simulink model "P3P_Grunert"  (R2023b)
settings: Solver=FixedStepDiscrete  StartTime=0.0  StopTime=0  RelTol=1e-3
values from neighbouring files (symbols this model uses):
  checkerSize = [5, 8]    [P3P_processVideo.m]
  checkerSquareLength = 31    [P3P_processVideo.m]
  I_current = I_allFrames(:,:,q)    [P3P_processVideo.m]
  K = [1109 0 640; 0 1109 360; 0 0 1]    [P3P_processVideo.m]
  x_pnts_i = round(x_pnts_i)    [P3P_processVideo.m]
  X_pnts_w = calcCheckerEdgeCoords_w(checkerSize, checkerSquareLength)    [P3P_processVideo.m]
undefined symbols (not defined in the file or in its folder): gray, Rec, SDTV
libraries: dspinverses x5, dspmathops x5, visiontextngfix x4, matrix_library x2, visionconversions x1, visionanalysis x1, dspvision x1, visionsources x1
(part 2 of 3)

== matlab function P3P_Grunert/While Iterator Subsystem/Perform P3P and RANSAC on checkerboard/Custom P3P solver (Grunert)/Find ray lengths jingnanshi convention ==
  data: l_AB input; soln output size=[4, 3]; l_BC input; l_AC input; theta input
function soln = fcn(l_AB, l_BC, l_AC, theta)

soln = zeros(4, 3);


%Calculate polynomial coefficients
a = l_AC;
b = l_BC;
c = l_AB;

gamma = theta(1); %theta_AB
alpha = theta(3); %theta_AC
beta = theta(2); %theta_BC


a2minc2ovb2 =  (a^2 - c^2) / b^2 ;
a2plusc2ovb2 =  (a^2 + c^2) / b^2; 


A0 = (1 + a2minc2ovb2)^2   -   4*((a*cos(gamma)/b)^2);
A1 = - a2minc2ovb2 * (1 + a2minc2ovb2) * cos(beta)     +    2 * ((a * cos(gamma) /  b)^2) * cos (beta)     -     (1 - a2plusc2ovb2) * cos(alpha) * cos(gamma);
A1 = 4 * A1;
A2 = a2minc2ovb2^2   -   1   +   2*((a2minc2ovb2 * cos(beta))^2)  +  2 *(  ((b^2 - c^2)/(b^2))  * (cos(alpha))^2  )   - 4*a2plusc2ovb2*cos(alpha)*cos(beta)*cos(gamma)   +   2*((b^2 - a^2)/(b^2))*((cos(gamma))^2);
A2 = 2* A2;
A3 = a2minc2ovb2 * (1 - a2minc2ovb2) * cos(beta)    -   (1 - a2plusc2ovb2) * cos(alpha) * cos(gamma)    +   2 * ((c * cos(alpha)/b)^2) * cos(beta);
A3 = 4 * A3;
A4 = (a2minc2ovb2 -1)^2   - (2 * c * cos(alpha) / b)^2;

%Solve polynomial
%instead of u and v for polynomial, use g and h - i.e., g = s2/s1 and h =
%s3/s1
p = [A4 A3 A2 A1 A0];
h = roots(p);
%choose only real roots - maybe this is not necessary?
h = h(imag(h)==0);
h = real(h);

%%%%%%%%%%%%%%%%%%%%%%%%%%%%%%%%%%%%%%%%%
%%%%%%%%%%%%%Find ray lengths

%For s1, which corresponds to sB. Should end up with 4 solns
%s_A =    (b^2) / (1 + h.^2  +  2*h*cos(beta)  )     ;
%s_A = s_A(s_A~=0);
%s_A = transpose(s_A);
%s_A = s_A.^0.5;


%Find s2, which corresponds to sC.
counter = 1
for i = 1:numel(h)

    s_1 = (b^2) / (1 + (h(i)^2) - 2*h(i)*cos(beta));
    s_1 = sqrt(s_1);

    G2 = s_1^2;
    G1 = - 2 * (s_1^2) * cos(gamma);
    G0 = (s_1^2 -c^2);

    g = roots([G2 G1 G0]);
    g = g(imag(g)==0);
    g = real(g);

    %First, solve for s_C, since it only depends on h and s_A:

    for j = 1:numel(g)
        soln(counter, 1) = s_1 * g(j);
        soln(counter, 3) = s_1 * h(i);
        soln(counter, 2) = s_1; 
        counter = counter +1
    end

end

== matlab function P3P_Grunert/While Iterator Subsystem/Perform P3P and RANSAC on checkerboard/Custom P3P solver (Grunert)/MATLAB Function4 ==
  data: pnts_vectorsCameraCoords input; theta_raysABC_radians output
function theta_raysABC_radians = calcProjectionRayAngles(pnts_vectorsCameraCoords)

A_x_c = pnts_vectorsCameraCoords(:,1);
B_x_c = pnts_vectorsCameraCoords(:,2);
C_x_c = pnts_vectorsCameraCoords(:,3);

%theta_AB = acos(dot(A_x_c, B_x_c));
%theta_BC = acos(dot(B_x_c, C_x_c));
%theta_AC = acos(dot(C_x_c, A_x_c));

%theta_AB = atan2(norm(cross(A_x_c, B_x_c)), dot(A_x_c, B_x_c));
%theta_BC = atan2(norm(cross(B_x_c, C_x_c)), dot(B_x_c, C_x_c));
%theta_AC = atan2(norm(cross(A_x_c, C_x_c)), dot(A_x_c, C_x_c)); 

theta_AB = acos(dot(A_x_c, B_x_c)/(norm(A_x_c)*norm(B_x_c)));
theta_BC = acos(dot(B_x_c, C_x_c)/(norm(B_x_c)*norm(C_x_c)));
theta_AC = acos(dot(A_x_c, C_x_c)/(norm(A_x_c)*norm(C_x_c)));


theta_raysABC_radians = [theta_AB; theta_BC; theta_AC];

== matlab function P3P_Grunert/While Iterator Subsystem/Perform P3P and RANSAC on checkerboard/Detect checkerboard corners ==
  data: x_pts_i output size=[60, 2]; I input; checkerSize output size=[1, 2]
function [x_pts_i, checkerSize]= findCheckerboardPnts(I)

%I = imread(fullfile('C:\Users\Alyssa\OneDrive - University of Cape Town\Vision\ESP32-CAM\CamCalibrationPics', '1.jpg'));
Points = detectCheckerboardPoints(I);
[~,checkerSize] = detectCheckerboardPoints(I);
x_pts_i = round(Points);
%checkerSize = Size;
%checkerPoints = imagePoints;

== matlab function P3P_Grunert/While Iterator Subsystem/Perform P3P and RANSAC on checkerboard/Extract best Rte (most inliers) ==
  data: Rte input; bestRt output; bestRt_error output; bestRt_inliers output
function [bestRt, bestRt_error, bestRt_inliers]= fcn(Rte)
%Function looks through 3-dim array Rte to find the Rt that has the highest
%number of inliers. This is output as the "best" Rt


index_bestRte = 0;
mostInliers = 0;

for n=1: size(Rte, 3)

    if Rte(1, 5, n) > mostInliers
        mostInliers = Rte(1, 5, n);
        index_bestRte = n;
    end
end

bestRt = Rte(:, 1:4, index_bestRte);
bestRt_error = Rte(2, 5, index_bestRte);
bestRt_inliers = Rte(1, 5, index_bestRte);

== matlab function P3P_Grunert/While Iterator Subsystem/Perform P3P and RANSAC on checkerboard/For Each Subsystem/Choose best solutiion from iteration ==
  data: Rt input; mostInliers_Rt output size=[3,4]; x_rem_i input; X_rem_w input; mostInliers output; Inlier_threshold input; mostInliers_avgError output; K input
function [mostInliers_Rt, mostInliers, mostInliers_avgError] = fcn(Rt, x_rem_i, X_rem_w, Inlier_threshold, K)
%This function finds the best Rt (transformation matrix) from the current
%RANSAC iteration. Here, "best" means "most inliers". I.e., for each 
%possible Rt out of the P3P solver, each of the remaining detected corners are 
%reprojected (using this Rt). If the reprojection error for a given point
%is below a certain threshold, it is considered an inlier. 
%Out of the 4 possible Rts for each P3P iteration, only that with the
%highest number of iterations will be passed out of this function.

%for each possible solution given by the P3P solver
numTestPts =  size(x_rem_i, 1);
mostInliers = 0;
mostInliers_Rt = zeros(3, 4);
mostInliers_avgError = 0;

for n = 1: size(Rt, 3)

    
    numInliers_n = 0;
    avgError_n = 0;

    %calculate reprojection error 
    for j = 1: numTestPts

        X_j_w = transpose(X_rem_w(j, :));
        x_j_i_real = transpose(x_rem_i(j,:));
        x_j_i_proj = zeros(2, 1);
        x_j_i_proj_homo = zeros(3,1);

        %project point (in homogenous coordinates)
        x_j_i_proj_homo = K * (  (Rt(:, 1:3, n) * X_j_w)  + Rt(:, 4,n)  );

        %Normalise by the 3rd dimension
        x_j_i_proj(1) = x_j_i_proj_homo(1)/x_j_i_proj_homo(3);
        x_j_i_proj(2) = x_j_i_proj_homo(2)/x_j_i_proj_homo(3);

        %calculate reprojection error for current point
        error_j = norm(x_j_i_proj - x_j_i_real);
        avgError_n = avgError_n + error_j;

        %check if an inlier
        if error_j < Inlier_threshold
            numInliers_n = numInliers_n + 1;
        end
    end
    
    %Calculate mean error (could be useful)
    avgError_n = avgError_n / numTestPts;

    %If current Rt achieves more inliers than previous best, then update
    %"best"
    if numInliers_n > mostInliers
        mostInliers = numInliers_n;
        mostInliers_avgError = avgError_n;
        mostInliers_Rt = Rt(:, :, n);
    end
end

== matlab function P3P_Grunert/While Iterator Subsystem/Perform P3P and RANSAC on checkerboard/For Each Subsystem/Create array ==
  data: Rte_n output size=[3,5]; mostInliers_Rt input; mostInliers input; mostInliers_avgError input
function Rte_n = fcn(mostInliers_Rt, mostInliers, mostInliers_avgError)

Rte_n = zeros(3, 5);
Rte_n(:, 1:4) = mostInliers_Rt;
Rte_n(1, 5) = mostInliers;
Rte_n(2, 5) = mostInliers_avgError;

== matlab function P3P_Grunert/While Iterator Subsystem/Perform P3P and RANSAC on checkerboard/For Each Subsystem/Custom P3P solver (Grunert)/Calc lengths of triangle sides (world frame) ==
  data: X_ABC_w input; l_AB output; l_BC output; l_AC output
function [l_AB, l_BC, l_AC]= fcn(X_ABC_w)

l_AB = norm(X_ABC_w(:,1)-X_ABC_w(:,2));
l_AC = norm(X_ABC_w(:,1)-X_ABC_w(:,3));
l_BC = norm(X_ABC_w(:,2)-X_ABC_w(:,3));

== matlab function P3P_Grunert/Subsystem/Custom P3P solver (Kneip)/Invert Rt (swap coord transformation)1 ==
  data: Rt input; Rt_converted output size=[3,4]
function Rt_converted = fcn(Rt)

R_inv = zeros(3,3);
t_inv = zeros(3,1);

R = Rt(1:3, 1:3);
t = Rt(1:3, 4);
  
R_inv(1:3, 1:3) = transpose(R);
t_inv = - R_inv * t;

%R_matlab_W = [-1 0 0; 0 1 0; 0 0 1];
%R_matlab_W = [-1 0 0; 0 -1 0; 0 0 1];
%R_conv = R_matlab_W * R_inv;
%t_conv = R_matlab_W * t_inv;

Rt_converted = [R_inv t_inv];

== matlab function P3P_Grunert/Subsystem/Custom P3P solver (Grunert)/Calculate rotation matrix and translation vector using SVD ==
  data: X_ABC_w input; Rt output size=[3,4,8]; X_ABC_c input
function Rt = fcn(X_ABC_w, X_ABC_c)

%We have 3 points in the world frame and in the camera frame. Now we need 
%to find the rotation and translation matrices that would convert one to 
%the other.
%This is the classic Procrustes problem, which we can solve using singular 
%value decomposition. We will end up with one rotation matrix and one
%translation vector for each of the possible sets of coordinates. 

 R = zeros(3,3,8);
 t = zeros(3,8);
 Rt = zeros(3,4,8);

 P = X_ABC_w;
 %Find the mean of the columns (i.e. the centroid of the shape)
 P_centroid = mean(P,2);
 %Centre each vector
 Q = P - P_centroid;

%for each possible solution
for i=1: size(X_ABC_c, 3)

    %Condition each vector as above
    P_dash =  X_ABC_c(:, :, i);
    P_dash_centroid = mean(P_dash, 2);
    Q_dash = P_dash - P_dash_centroid;
    
    %Find the covariance matrix
    H = Q_dash * transpose(Q);

    %Perform SVD (singular value decomposition)
    [U, S, V] = svd(H);

    % %Calculate rotation matrix
    R(:,:,i) = U * transpose(V);
    %Correct sign if needed
    if det(R(:,:,i))<0
        U(:,end) = -1 * U(:,end);
        %and recompute R
        R(:, :, i) = U * transpose(V);
    end

    % R(:,:,i) = transpose(U) * V;
    % if det(R(:,:,i)) < 0
    %     V(:,end) = -V(:,end);
    %     R = transpose(U) * V;
    % end

    %Calculate the translation vector:
    t(:, i) = P_dash_centroid - R(:, :, i)*P_centroid;

    Rt(:,:, i)= [R(:,:,i) t(:, i)];

end

== matlab function P3P_Grunert/While Iterator Subsystem/Perform P3P and RANSAC on checkerboard/For Each Subsystem/Custom P3P solver (Grunert)/Calculate rotation matrix and translation vector using SVD ==
  data: X_ABC_w input; Rt output size=[3,4,8]; X_ABC_c input
function Rt = fcn(X_ABC_w, X_ABC_c)

%We have 3 points in the world frame and in the camera frame. Now we need 
%to find the rotation and translation matrices that would convert one to 
%the other.
%This is the classic Procrustes problem, which we can solve using singular 
%value decomposition. We will end up with one rotation matrix and one
%translation vector for each of the possible sets of coordinates. 

 R = zeros(3,3,8);
 t = zeros(3,8);
 Rt = zeros(3,4,8);

 P = X_ABC_w;
 %Find the mean of the columns (i.e. the centroid of the shape)
 P_centroid = mean(P,2);
 %Centre each vector
 Q = P - P_centroid;

%for each possible solution
for i=1: size(X_ABC_c, 3)

    %Condition each vector as above
    P_dash =  X_ABC_c(:, :, i);
    P_dash_centroid = mean(P_dash, 2);
    Q_dash = P_dash - P_dash_centroid;
    
    %Find the covariance matrix
    H = Q_dash * transpose(Q);

    %Perform SVD (singular value decomposition)
    [U, S, V] = svd(H);

    %Calculate rotation matrix
    R(:,:,i) = U * transpose(V);
    %Correct sign if needed
    if det(R(:,:,i))<0
        U(:,end) = U(:,end) * (-1);
        %and recompute R
        R(:, :, i) = U * transpose(V);
    end

    %Calculate the translation vector:
    t(:, i) = P_dash_centroid - R(:, :, i)*P_centroid;

    Rt(:,:, i)= [R(:,:,i) t(:, i)];

end

== matlab function P3P_Grunert/Subsystem/Custom P3P solver (Kneip)/Invert Rt (swap coord transformation)2 ==
  data: Rt input; Rt_converted output size=[3,4]
function Rt_converted = fcn(Rt)

R_inv = zeros(3,3);

R = Rt(1:3, 1:3);
t = Rt(1:3, 4);
  
R_inv(1:3, 1:3) = transpose(R);
t_inv = - R_inv * t;

%R_matlab_W = [-1 0 0; 0 1 0; 0 0 1];
%R_matlab_W = [-1 0 0; 0 -1 0; 0 0 1];
%R_conv = R_matlab_W * R_inv;
%t_conv = R_matlab_W * t_inv;

Rt_converted = [R_inv t_inv];

== matlab function P3P_Grunert/While Iterator Subsystem/Perform P3P and RANSAC on checkerboard/For Each Subsystem/Custom P3P solver (Grunert)/Compute 3D coords of control points A, B, C in camera coord system ==
  data: s_ABC input; X_c_ABC output size=[3,3,8]; x_c_norm_ABC input
function X_c_ABC = fcn(s_ABC, x_c_norm_ABC)
    X_c_ABC = zeros(3,3,8);


    %For each combination of possible lengths
    for n=1:size(s_ABC, 1)
        %Get the vector between the camera and the point by multiplying
        %each element of the (unit) direction vector with the associated
        %ray length from the solution. 
        %The solution takes the form: [s_A1 s_B1 s_C1; s_A2 sB2...].
        %The direction vectors take the form: [xA xB xC; yA yB...].
        X_c_ABC(:, 1, n) = s_ABC(n, 1) * x_c_norm_ABC(:, 1);
        X_c_ABC(:, 2, n) = s_ABC(n, 2) * x_c_norm_ABC(:, 2);
        X_c_ABC(:, 3, n) = s_ABC(n, 3) * x_c_norm_ABC(:, 3);
    end

== matlab function P3P_Grunert/While Iterator Subsystem/Perform P3P and RANSAC on checkerboard/For Each Subsystem/Custom P3P solver (Grunert)/Find ray lengths ==
  data: l_AB input; soln output size=[4, 3]; l_BC input; l_AC input; theta input
function soln = fcn(l_AB, l_BC, l_AC, theta)

soln = zeros(4, 3);


%Calculate polynomial coefficients
a = l_BC;
b = l_AC;
c = l_AB;

gamma = theta(3); %theta_AC
alpha = theta(2); %theta_BC
beta = theta(1); %theta_AB


a2minc2ovb2 =  (a^2 - c^2) / b^2 ;
a2plusc2ovb2 =  (a^2 + c^2) / b^2; 


A0 = (1 + a2minc2ovb2)^2   -   4*((a*cos(gamma)/b)^2);
A1 = - a2minc2ovb2 * (1 + a2minc2ovb2) * cos(beta)     +    2 * ((a * cos(gamma) /  b)^2) * cos (beta)     -     (1 - a2plusc2ovb2) * cos(alpha) * cos(gamma);
A1 = 4 * A1;
A2 = a2minc2ovb2^2   -   1   +   2*((a2minc2ovb2 * cos(beta))^2)  +  2 *(  ((b^2 - c^2)/(b^2))  * (cos(alpha))^2  )   - 4*a2plusc2ovb2*cos(alpha)*cos(beta)*cos(gamma)   +   2*((b^2 - a^2)/(b^2))*(cos(gamma)^2);
A2 = 2* A2;
A3 = a2minc2ovb2 * (1 - a2minc2ovb2) * cos(beta)    -   (1 - a2plusc2ovb2) * cos(alpha) * cos(gamma)    +   2 * ((c * cos(alpha)/b)^2) * cos(beta);
A3 = 4 * A3;
A4 = (a2minc2ovb2 -1)^2   - (2 * c * cos(alpha) / b)^2;

%Solve polynomial
%instead of u and v for polynomial, use g and h - i.e., g = s2/s1 and h =
%s3/s1
p = [A4 A3 A2 A1 A0];
h = roots(p);
%choose only real roots - maybe this is not necessary?
h = h(imag(h)==0);
h = real(h);

%%%%%%%%%%%%%%%%%%%%%%%%%%%%%%%%%%%%%%%%%
%%%%%%%%%%%%%Find ray lengths

%For s1, which corresponds to sA. Should end up with 4 solns
%s_A =    (b^2) / (1 + h.^2  +  2*h*cos(beta)  )     ;
%s_A = s_A(s_A~=0);
%s_A = transpose(s_A);
%s_A = s_A.^0.5;


%Find s2, which corresponds to sC.
counter = 1
for i = 1:numel(h)

    s_A = (b^2) / (1 + (h(i)^2) - 2*h(i)*cos(beta));
    s_A = sqrt(s_A);

    G2 = s_A^2;
    G1 = - 2 * (s_A^2) * cos(gamma);
    G0 = (s_A -c)^2;

    g = roots([G2 G1 G0]);
    g = g(imag(g)==0);
    g = real(g);

    %First, solve for s_C, since it only depends on h and s_A:

    for j = 1:numel(g)
        soln(counter, 1) = s_A;
        soln(counter, 3) = s_A * g(j);
        soln(counter, 2) = h(i) * s_A;
        counter = counter +1
    end

end

== matlab function P3P_Grunert/While Iterator Subsystem/Perform P3P and RANSAC on checkerboard/For Each Subsystem/Custom P3P solver (Grunert)/Find ray lengths jingnanshi convention ==
  data: l_AB input; soln output size=[8, 3]; l_BC input; l_AC input; theta input
function soln = fcn(l_AB, l_BC, l_AC, theta)

soln = zeros(8, 3);


%Calculate polynomial coefficients
a = l_AC;
b = l_BC;
c = l_AB;

gamma = theta(1); %theta_AB
alpha = theta(3); %theta_AC
beta = theta(2); %theta_BC


a2minc2ovb2 =  (a^2 - c^2) / b^2 ;
a2plusc2ovb2 =  (a^2 + c^2) / b^2; 


A0 = (1 + a2minc2ovb2)^2   -   4*((a*cos(gamma)/b)^2);
A1 = - a2minc2ovb2 * (1 + a2minc2ovb2) * cos(beta)     +    2 * ((a * cos(gamma) /  b)^2) * cos (beta)     -     (1 - a2plusc2ovb2) * cos(alpha) * cos(gamma);
A1 = 4 * A1;
A2 = a2minc2ovb2^2   -   1   +   2*((a2minc2ovb2 * cos(beta))^2)  +  2 *(  ((b^2 - c^2)/(b^2))  * (cos(alpha))^2  )   - 4*a2plusc2ovb2*cos(alpha)*cos(beta)*cos(gamma)   +   2*((b^2 - a^2)/(b^2))*((cos(gamma))^2);
A2 = 2* A2;
A3 = a2minc2ovb2 * (1 - a2minc2ovb2) * cos(beta)    -   (1 - a2plusc2ovb2) * cos(alpha) * cos(gamma)    +   2 * ((c * cos(alpha)/b)^2) * cos(beta);
A3 = 4 * A3;
A4 = (a2minc2ovb2 -1)^2   - (2 * c * cos(alpha) / b)^2;

%Solve polynomial
%instead of u and v for polynomial, use g and h - i.e., g = s2/s1 and h =
%s3/s1
p = [A4 A3 A2 A1 A0];
h = roots(p);
%choose only real roots - maybe this is not necessary?
h = h(imag(h)==0);
h = real(h);

%%%%%%%%%%%%%%%%%%%%%%%%%%%%%%%%%%%%%%%%%
%%%%%%%%%%%%%Find ray lengths

%For s1, which corresponds to sB. Should end up with 4 solns
%s_A =    (b^2) / (1 + h.^2  +  2*h*cos(beta)  )     ;
%s_A = s_A(s_A~=0);
%s_A = transpose(s_A);
%s_A = s_A.^0.5;


%Find s2, which corresponds to sC.
counter = 1;
for i = 1:numel(h)

    s_1 = (b^2) / (1 + (h(i)^2) - 2*h(i)*cos(beta));
    s_1 = sqrt(s_1);

    G2 = s_1^2;
    G1 = - 2 * (s_1^2) * cos(gamma);
    G0 = (s_1^2 -c^2);

    g = roots([G2 G1 G0]);
    g = g(imag(g)==0);
    g = real(g);

    %First, solve for s_C, since it only depends on h and s_A:

    for j = 1:numel(g)
        soln(counter, 1) = s_1 * g(j);
        soln(counter, 3) = s_1 * h(i);
        soln(counter, 2) = s_1; 
        counter = counter +1;
    end

end

== matlab function P3P_Grunert/While Iterator Subsystem/Perform P3P and RANSAC on checkerboard/For Each Subsystem/Custom P3P solver (Grunert)/MATLAB Function4 ==
  data: pnts_vectorsCameraCoords input; theta_raysABC_radians output
function theta_raysABC_radians = calcProjectionRayAngles(pnts_vectorsCameraCoords)

A_x_c = pnts_vectorsCameraCoords(:,1);
B_x_c = pnts_vectorsCameraCoords(:,2);
C_x_c = pnts_vectorsCameraCoords(:,3);

%theta_AB = acos(dot(A_x_c, B_x_c));
%theta_BC = acos(dot(B_x_c, C_x_c));
%theta_AC = acos(dot(C_x_c, A_x_c));

%theta_AB = atan2(norm(cross(A_x_c, B_x_c)), dot(A_x_c, B_x_c));
%theta_BC = atan2(norm(cross(B_x_c, C_x_c)), dot(B_x_c, C_x_c));
%theta_AC = atan2(norm(cross(A_x_c, C_x_c)), dot(A_x_c, C_x_c)); 

theta_AB = acos(dot(A_x_c, B_x_c)/(norm(A_x_c)*norm(B_x_c)));
theta_BC = acos(dot(B_x_c, C_x_c)/(norm(B_x_c)*norm(C_x_c)));
theta_AC = acos(dot(A_x_c, C_x_c)/(norm(A_x_c)*norm(C_x_c)));


theta_raysABC_radians = [theta_AB; theta_BC; theta_AC];

== matlab function P3P_Grunert/While Iterator Subsystem/Perform P3P and RANSAC on checkerboard/For Each Subsystem/extract P3P points and remove them from point matrices ==
  data: Vec_iterations input; x_ABC_i output size=[2,3]; X_pts_w input; X_ABC_w output size=[3,3]; x_pts_i input; x_rem_i output size=[60, 2]; X_rem_w output size=[60, 3]
function [x_ABC_i, X_ABC_w, x_rem_i, X_rem_w]= fcn(Vec_iterations, X_pts_w, x_pts_i)

num_pts = size(x_pts_i, 1);

%Initialise variables
rng("shuffle");
randNum1 = randi(num_pts);
randNum2 = randi(num_pts);
randNum3 = randi(num_pts);
while (randNum2 == randNum1)
    randNum2 = randi(num_pts);
end

while ((randNum3 ==randNum2) || (randNum3 == randNum1))
    randNum3 = randi(num_pts);
end
pnt1 = [X_pts_w(randNum1, :) x_pts_i(randNum1, :)];
pnt2 = [X_pts_w(randNum2, :) x_pts_i(randNum2, :)];
pnt3 = [X_pts_w(randNum3, :) x_pts_i(randNum3, :)];

%Choose random points  - sample until their x and y values are unique
% while (pnt1(1,1)==pnt2(1,1) || pnt1(1,1)==pnt3(1,1) || pnt2(1,1)==pnt3(1,1)) || (pnt1(1,2)==pnt2(1,2) || pnt1(1,2)==pnt3(1,2) || pnt2(1,2)==pnt3(1,2))
%     rng("shuffle");
%     randNum1 = randi(num_pts)
%     randNum2 = randi(num_pts)
%     randNum3 = randi(num_pts)
%     pnt1 = [X_pts_w(randNum1, :) x_pts_i(randNum1, :)];
%     pnt2 = [X_pts_w(randNum2, :) x_pts_i(randNum2, :)];
%     pnt3 = [X_pts_w(randNum3, :) x_pts_i(randNum3, :)];
% 
% end




%Force select the corner points
%randNums = [1 6 49];
%pnt1 = [X_pts_w(randNums(1, 1), :) x_pts_i(randNums(1, 1), :)];
%pnt2 = [X_pts_w(randNums(1, 2), :) x_pts_i(randNums(1, 2), :)];
%pnt3 = [X_pts_w(randNums(1, 3), :) x_pts_i(randNums(1, 3), :)];

%Remove training points from the list - i.e., develop "verification" set
X_rem_w = X_pts_w;
%X_rem_w((randNums(1)), :) = [];
%X_rem_w((randNums(2)-1), :) = [];
%X_rem_w((randNums(3)-2), :) = [];

x_rem_i = x_pts_i;
%x_rem_i(randNums(1), :) = [];
%x_rem_i((randNums(2)-1), :) = [];
%x_rem_i((randNums(3)-2), :) = [];


%Must put the points "in order" - is this necessary? Not sure. Early
%results suggest that it might be.
X_train = [pnt1; pnt2; pnt3];
X_train =sortrows(X_train, 2);          %sort by y-coordinate (world)
X_train_sorted = X_train;
%Swap rows
if X_train(2, 1) > X_train(3, 1)
    X_train_sorted([2 3], :) = X_train([3 2], :);
end

X_A_w = X_train_sorted(1, 1:3);
X_B_w = X_train_sorted(2, 1:3);
X_C_w = X_train_sorted(3, 1:3);

x_A_i = X_train_sorted(1, 4:5);
x_B_i = X_train_sorted(2, 4:5);
x_C_i = X_train_sorted(3, 4:5);

X_ABC_w_vert = [X_A_w; X_B_w; X_C_w];
X_ABC_w = transpose(X_ABC_w_vert);

x_ABC_i_vert = [x_A_i; x_B_i; x_C_i];
x_ABC_i = transpose(x_ABC_i_vert);

== matlab function P3P_Grunert/While Iterator Subsystem/Perform P3P and RANSAC on checkerboard/Image size calculator (in pixels) ==
  data: imageMatrix input; imageSize output
function imageSize = fcn(imageMatrix)

imageSize = [size(imageMatrix, 1) size(imageMatrix,2)];

== matlab function P3P_Grunert/While Iterator Subsystem/Perform P3P and RANSAC on checkerboard/MATLAB P3P solver1 ==
  data: estTransform input; K input; imagePts input; worldPts input; imageSize input; A output
function A = fcn(estTransform, K, imagePts, worldPts, imageSize)

    %imagePts_vert = transpose(imagePts);
    %worldPts_vert = transpose(worldPts);
    focalLngth = [K(1,1) K(2,2)];
    principalPnt = [K(1,3) K(2,3)];

    coder.extrinsic('builtinP3P');
    A = zeros(4,4);

    
    estTransform_R_inv = inv(estTransform(:, 1:3));
    estTransform_negTranslation_Rotated = estTransform_R_inv * (-estTransform(:, 4));

    A = builtinP3P(imagePts, worldPts, focalLngth, principalPnt, imageSize, estTransform_negTranslation_Rotated, estTransform_R_inv);

    %intr = cameraIntrinsics(focalLngth, principalPnt, imageSize)

    %worldPose = estworldpose(imagePts_vert, worldPts_vert, intr)

    %pcshow(worldPts,VerticalAxis="Y",VerticalAxisDir="down", ...
    %MarkerSize=30);
    %hold on
    %plotCamera(Size=10,Orientation=worldPose.R', ...
    %    Location=worldPose.Translation);
    %hold off

== matlab function P3P_Grunert/Subsystem/Custom P3P solver (Grunert)/Compute 3D coords of control points A, B, C in camera coord system ==
  data: s_ABC input; X_c_ABC output size=[3,3,8]; x_c_norm_ABC input
function X_c_ABC = fcn(s_ABC, x_c_norm_ABC)
    X_c_ABC = zeros(3,3,8);


    %For each combination of possible lengths
    for n=1:size(s_ABC, 1)
        %Get the vector between the camera and the point by multiplying
        %each element of the (unit) direction vector with the associated
        %ray length from the solution. 
        %The solution takes the form: [s_A1 s_B1 s_C1; s_A2 sB2...].
        %The direction vectors take the form: [xA xB xC; yA yB...].
        X_c_ABC(:, 1, n) = s_ABC(n, 1) * x_c_norm_ABC(:, 1);
        X_c_ABC(:, 2, n) = s_ABC(n, 2) * x_c_norm_ABC(:, 2);
        X_c_ABC(:, 3, n) = s_ABC(n, 3) * x_c_norm_ABC(:, 3);
    end

== matlab function P3P_Grunert/While Iterator Subsystem/Perform P3P and RANSAC on checkerboard/Outer corner selectors/MATLAB Function ==
  data: boardSize input; B_index output; C_index output; D_index output
function [B_index, C_index, D_index]= fcn(boardSize)

B_index = boardSize(1) - 1;
C_index = ((boardSize(1) - 1) * (boardSize(2) - 2)) + 1;
D_index = ((boardSize(1) - 1) * (boardSize(2) - 1)) ;

== matlab function P3P_Grunert/While Iterator Subsystem/Perform P3P and RANSAC on checkerboard/Outer corner selectors/Outer corner selector ==
  data: x_ABC_i output; x_D_i output; pntMatrix input; A_index input; B_index input; C_index input; D_index input
function [x_ABC_i, x_D_i] = calcPntVectors_PrincipalPntToImagePlane(pntMatrix, A_index, B_index, C_index, D_index)

%Obtain pixel positions
A_u = pntMatrix(A_index,1);
A_v = pntMatrix(A_index,2);

B_u = pntMatrix(B_index, 1);
B_v = pntMatrix(B_index, 2);

C_u = pntMatrix( C_index , 1);
C_v = pntMatrix( C_index , 2);

D_u = pntMatrix( D_index, 1);
D_v = pntMatrix(D_index, 2);


%Created augmented U matrices - i.e., add extra row of "1"
x_ABC_i = [A_u B_u C_u; A_v B_v C_v]
%pnts_U_ABC_aug = [pnts_U_ABC; 1 1 1];

%pnts_X_c = inv(K) * pnts_U_ABC_aug;

%pntVectors_cameraCoords = pnts_X_c;
%pntsABC_imageCoords = pnts_U_ABC;
%pntsABCD_imageCoords = [A_u B_u C_u D_u; A_v B_v C_v D_v];
x_D_i = [D_u; D_v];

== matlab function P3P_Grunert/While Iterator Subsystem/Perform P3P and RANSAC on checkerboard/Outer corner selectors/Outer corner selector (world frame) ==
  data: X_Pts_w input; X_ABC_w output size=[3, 3]; X_D_w output size=[3, 1]; A_index input; B_index input; C_index input; D_index input
function [X_ABC_w, X_D_w]= calcPtoPLengths_world(X_Pts_w, A_index, B_index, C_index, D_index)
    
    X_A_w = X_Pts_w(A_index, :);
    X_B_w = X_Pts_w(B_index, :);
    X_C_w = X_Pts_w(C_index, :);
    X_D_w_vert = X_Pts_w(D_index, :);

    X_ABC_w_vert = [X_A_w; X_B_w; X_C_w];
    X_ABC_w = transpose(X_ABC_w_vert);
    X_D_w = transpose(X_D_w_vert);

== matlab function P3P_Grunert/While Iterator Subsystem/Perform P3P and RANSAC on checkerboard/Project 4th point and calc reprojection error ==
  data: Rt input; K input; X_D_w input; x_D_i input; x_D_i_proj output size=[2,4]; soln output size=[3,4]; min_error output
function [x_D_i_proj, soln, min_error]= fcn(Rt, K, X_D_w, x_D_i)

%Calculate the projection of a fourth point onto the image plane, based on 
%the candidate rotation matrices and translation vectors. Later, we
%will check how well this corresponds with where it was actually observed.
    
    %Initialise vector
    x_D_i_proj = zeros(2,4); %where i stands for "image plane"
    x_D_i_proj_homo = zeros(3,4); %where i stands for "image plane"
    error = zeros(1,4);     %reprojection error
    soln = zeros(3, 4);

    %For each possible solution
    for n=1: size(Rt, 3)

        %Calculate projection of the point D
        x_D_i_proj_homo(:, n) = K * (  (Rt(:, 1:3, n) * X_D_w)  + Rt(:, 4,n)  );

        %Normalise by the 3rd dimension
        x_D_i_proj(1,n) = x_D_i_proj_homo(1,n)/x_D_i_proj_homo(3,n);
        x_D_i_proj(2,n) = x_D_i_proj_homo(2,n)/x_D_i_proj_homo(3,n);

        %Calculate reprojection error
        error(1, n) = norm(x_D_i - x_D_i_proj(:, n));
    
    end

    %Choose lower reprojection error
    error(1, 1) = norm(x_D_i - x_D_i_proj(:, 1));
    min_error = error(1,1);
    soln = Rt(:, :, 1);
    
    for j=2 : size(x_D_i_proj, 2)
        
        if error(1, j) < min_error
            min_error = error(1, j);
            soln = Rt(:, :, j);
        end
    
    end

== matlab function P3P_Grunert/Calc coords of all control points in world frame ==
  data: X_pts_w output size=[60, 3]; checkerSize input; squareEdgeLength input
function X_pts_w = calcPtoPLengths_world(checkerSize, squareEdgeLength)
    
    boardWidth = checkerSize(2);
    boardHeight = checkerSize(1);
    X_pts_w = zeros((boardWidth-1)*(boardHeight-1), 3);

    %for each column
    for c=1 : boardWidth-1
        for r = 1: boardHeight-1
            x = (c-1)*squareEdgeLength;
            y = (r-1)*squareEdgeLength;
            z = 0;
            X_pts_w(  (((c-1)*(boardHeight-1)) + r), 1) = x;
            X_pts_w(  (((c-1)*(boardHeight-1)) + r), 2) = y;
            X_pts_w(  (((c-1)*(boardHeight-1)) + r), 3) = z;
        end
    end

== matlab function P3P_Grunert/Detect checkerboard corners ==
  data: x_pts_i output size=[60, 2]; I input; checkerSize output size=[1, 2]
function [x_pts_i, checkerSize]= findCheckerboardPnts(I)

%I = imread(fullfile('C:\Users\Alyssa\OneDrive - University of Cape Town\Vision\ESP32-CAM\CamCalibrationPics', '1.jpg'));
Points = detectCheckerboardPoints(I);
[~,checkerSize] = detectCheckerboardPoints(I);
x_pts_i = round(Points);
%checkerSize = Size;
%checkerPoints = imagePoints;

== matlab function P3P_Grunert/Subsystem/Extract best Rte (most inliers) ==
  data: Rte input; bestRt output; bestRt_error output; bestRt_inliers output
function [bestRt, bestRt_error, bestRt_inliers]= fcn(Rte)
%Function looks through 3-dim array Rte to find the Rt that has the highest
%number of inliers. This is output as the "best" Rt


index_bestRte = 0;
mostInliers = 0;

for n=1: size(Rte, 3)

    if Rte(1, 5, n) > mostInliers
        mostInliers = Rte(1, 5, n);
        index_bestRte = n;
    end
end

bestRt = Rte(:, 1:4, index_bestRte);
bestRt_error = Rte(2, 5, index_bestRte);
bestRt_inliers = Rte(1, 5, index_bestRte);

== matlab function P3P_Grunert/Subsystem/For Each Subsystem/Choose best solutiion from iteration ==
  data: Rt input; mostInliers_Rt output size=[3,4]; x_rem_i input; X_rem_w input; mostInliers output; Inlier_threshold input; mostInliers_avgError output; K input
function [mostInliers_Rt, mostInliers, mostInliers_avgError] = fcn(Rt, x_rem_i, X_rem_w, Inlier_threshold, K)
%This function finds the best Rt (transformation matrix) from the current
%RANSAC iteration. Here, "best" means "most inliers". I.e., for each 
%possible Rt out of the P3P solver, each of the remaining detected corners are 
%reprojected (using this Rt). If the reprojection error for a given point
%is below a certain threshold, it is considered an inlier. 
%Out of the 4 possible Rts for each P3P iteration, only that with the
%highest number of iterations will be passed out of this function.

%for each possible solution given by the P3P solver
numTestPts =  size(x_rem_i, 1);
mostInliers = 0;
mostInliers_Rt = zeros(3, 4);
mostInliers_avgError = 0;

for n = 1: size(Rt, 3)

    
    numInliers_n = 0;
    avgError_n = 0;

    %calculate reprojection error 
    for j = 1: numTestPts

        X_j_w = transpose(X_rem_w(j, :));
        x_j_i_real = transpose(x_rem_i(j,:));
        x_j_i_proj = zeros(2, 1);
        x_j_i_proj_homo = zeros(3,1);

        %project point (in homogenous coordinates)
        x_j_i_proj_homo = K * (  (Rt(:, 1:3, n) * X_j_w)  + Rt(:, 4,n)  );

        %Normalise by the 3rd dimension
        x_j_i_proj(1) = x_j_i_proj_homo(1)/x_j_i_proj_homo(3);
        x_j_i_proj(2) = x_j_i_proj_homo(2)/x_j_i_proj_homo(3);

        %calculate reprojection error for current point
        error_j = norm(x_j_i_proj - x_j_i_real);
        avgError_n = avgError_n + error_j;

        %check if an inlier
        if error_j < Inlier_threshold
            numInliers_n = numInliers_n + 1;
        end
    end
    
    %Calculate mean error (could be useful)
    avgError_n = avgError_n / numTestPts;

    %If current Rt achieves more inliers than previous best, then update
    %"best"
    if numInliers_n > mostInliers
        mostInliers = numInliers_n;
        mostInliers_avgError = avgError_n;
        mostInliers_Rt = Rt(:, :, n);
    end
end

== matlab function P3P_Grunert/Formulate intrinsics (hard-coded) ==
  data: K output; principalPnt output
function [K, principalPnt]= intrinsics

    fx = 1274.58238813250;
    fy = 1273.36371905619;
    Ox = 627.693937913345;
    Oy = 405.441250468717;

    K = [fx 0 Ox; 0 fy Oy; 0 0 1];

    principalPnt = [627.693937913345; 405.441250468717];

== matlab function P3P_Grunert/Subsystem/For Each Subsystem/Create array ==
  data: Rte_n output size=[3,5]; mostInliers_Rt input; mostInliers input; mostInliers_avgError input
function Rte_n = fcn(mostInliers_Rt, mostInliers, mostInliers_avgError)

Rte_n = zeros(3, 5);
Rte_n(:, 1:4) = mostInliers_Rt;
Rte_n(1, 5) = mostInliers;
Rte_n(2, 5) = mostInliers_avgError;

== matlab function P3P_Grunert/Subsystem/For Each Subsystem/Custom P3P solver (Grunert)/Calc lengths of triangle sides (world frame) ==
  data: X_ABC_w input; l_AB output; l_BC output; l_AC output
function [l_AB, l_BC, l_AC]= fcn(X_ABC_w)

l_AB = norm(X_ABC_w(:,1)-X_ABC_w(:,2));
l_AC = norm(X_ABC_w(:,1)-X_ABC_w(:,3));
l_BC = norm(X_ABC_w(:,2)-X_ABC_w(:,3));

== matlab function P3P_Grunert/Subsystem/For Each Subsystem/Custom P3P solver (Grunert)/Calculate rotation matrix and translation vector using SVD ==
  data: X_ABC_w input; Rt output size=[3,4,8]; X_ABC_c input
function Rt = fcn(X_ABC_w, X_ABC_c)

%We have 3 points in the world frame and in the camera frame. Now we need 
%to find the rotation and translation matrices that would convert one to 
%the other.
%This is the classic Procrustes problem, which we can solve using singular 
%value decomposition. We will end up with one rotation matrix and one
%translation vector for each of the possible sets of coordinates. 

 R = zeros(3,3,8);
 t = zeros(3,8);
 Rt = zeros(3,4,8);

 P = X_ABC_w;
 %Find the mean of the columns (i.e. the centroid of the shape)
 P_centroid = mean(P,2);
 %Centre each vector
 Q = P - P_centroid;

%for each possible solution
for i=1: size(X_ABC_c, 3)

    %Condition each vector as above
    P_dash =  X_ABC_c(:, :, i);
    P_dash_centroid = mean(P_dash, 2);
    Q_dash = P_dash - P_dash_centroid;
    
    %Find the covariance matrix
    H = Q_dash * transpose(Q);

    %Perform SVD (singular value decomposition)
    [U, S, V] = svd(H);

    % %Calculate rotation matrix
    R(:,:,i) = U * transpose(V);
    %Correct sign if needed
    if det(R(:,:,i))<0
        U(:,end) = -1 * U(:,end);
        %and recompute R
        R(:, :, i) = U * transpose(V);
    end

    % R(:,:,i) = transpose(U) * V;
    % if det(R(:,:,i)) < 0
    %     V(:,end) = -V(:,end);
    %     R = transpose(U) * V;
    % end

    %Calculate the translation vector:
    t(:, i) = P_dash_centroid - R(:, :, i)*P_centroid;

    Rt(:,:, i)= [R(:,:,i) t(:, i)];

end

== matlab function P3P_Grunert/Subsystem/For Each Subsystem/Custom P3P solver (Grunert)/Compute 3D coords of control points A, B, C in camera coord system ==
  data: s_ABC input; X_c_ABC output size=[3,3,8]; x_c_norm_ABC input
function X_c_ABC = fcn(s_ABC, x_c_norm_ABC)
    X_c_ABC = zeros(3,3,8);


    %For each combination of possible lengths
    for n=1:size(s_ABC, 1)
        %Get the vector between the camera and the point by multiplying
        %each element of the (unit) direction vector with the associated
        %ray length from the solution. 
        %The solution takes the form: [s_A1 s_B1 s_C1; s_A2 sB2...].
        %The direction vectors take the form: [xA xB xC; yA yB...].
        X_c_ABC(:, 1, n) = s_ABC(n, 1) * x_c_norm_ABC(:, 1);
        X_c_ABC(:, 2, n) = s_ABC(n, 2) * x_c_norm_ABC(:, 2);
        X_c_ABC(:, 3, n) = s_ABC(n, 3) * x_c_norm_ABC(:, 3);
    end

== matlab function P3P_Grunert/Subsystem/For Each Subsystem/Custom P3P solver (Grunert)/Find ray lengths ==
  data: l_AB input; soln output size=[4, 3]; l_BC input; l_AC input; theta input
function soln = fcn(l_AB, l_BC, l_AC, theta)

soln = zeros(4, 3);


%Calculate polynomial coefficients
a = l_BC;
b = l_AC;
c = l_AB;

gamma = theta(3); %theta_AC
alpha = theta(2); %theta_BC
beta = theta(1); %theta_AB


a2minc2ovb2 =  (a^2 - c^2) / b^2 ;
a2plusc2ovb2 =  (a^2 + c^2) / b^2; 


A0 = (1 + a2minc2ovb2)^2   -   4*((a*cos(gamma)/b)^2);
A1 = - a2minc2ovb2 * (1 + a2minc2ovb2) * cos(beta)     +    2 * ((a * cos(gamma) /  b)^2) * cos (beta)     -     (1 - a2plusc2ovb2) * cos(alpha) * cos(gamma);
A1 = 4 * A1;
A2 = a2minc2ovb2^2   -   1   +   2*((a2minc2ovb2 * cos(beta))^2)  +  2 *(  ((b^2 - c^2)/(b^2))  * (cos(alpha))^2  )   - 4*a2plusc2ovb2*cos(alpha)*cos(beta)*cos(gamma)   +   2*((b^2 - a^2)/(b^2))*(cos(gamma)^2);
A2 = 2* A2;
A3 = a2minc2ovb2 * (1 - a2minc2ovb2) * cos(beta)    -   (1 - a2plusc2ovb2) * cos(alpha) * cos(gamma)    +   2 * ((c * cos(alpha)/b)^2) * cos(beta);
A3 = 4 * A3;
A4 = (a2minc2ovb2 -1)^2   - (2 * c * cos(alpha) / b)^2;

%Solve polynomial
%instead of u and v for polynomial, use g and h - i.e., g = s2/s1 and h =
%s3/s1
p = [A4 A3 A2 A1 A0];
h = roots(p);
%choose only real roots - maybe this is not necessary?
h = h(imag(h)==0);
h = real(h);

%%%%%%%%%%%%%%%%%%%%%%%%%%%%%%%%%%%%%%%%%
%%%%%%%%%%%%%Find ray lengths

%For s1, which corresponds to sA. Should end up with 4 solns
%s_A =    (b^2) / (1 + h.^2  +  2*h*cos(beta)  )     ;
%s_A = s_A(s_A~=0);
%s_A = transpose(s_A);
%s_A = s_A.^0.5;


%Find s2, which corresponds to sC.
counter = 1
for i = 1:numel(h)

    s_A = (b^2) / (1 + (h(i)^2) - 2*h(i)*cos(beta));
    s_A = sqrt(s_A);

    G2 = s_A^2;
    G1 = - 2 * (s_A^2) * cos(gamma);
    G0 = (s_A -c)^2;

    g = roots([G2 G1 G0]);
    g = g(imag(g)==0);
    g = real(g);

    %First, solve for s_C, since it only depends on h and s_A:

    for j = 1:numel(g)
        soln(counter, 1) = s_A;
        soln(counter, 3) = s_A * g(j);
        soln(counter, 2) = h(i) * s_A;
        counter = counter +1
    end

end

== matlab function P3P_Grunert/Subsystem/For Each Subsystem/Custom P3P solver (Grunert)/Find ray lengths jingnanshi convention ==
  data: l_AB input; soln output size=[8, 3]; l_BC input; l_AC input; theta input
function soln = fcn(l_AB, l_BC, l_AC, theta)

soln = zeros(8, 3);


%Calculate polynomial coefficients
a = l_AC;
b = l_BC;
c = l_AB;

gamma = theta(1); %theta_AB
alpha = theta(3); %theta_AC
beta = theta(2); %theta_BC


a2minc2ovb2 =  (a^2 - c^2) / b^2 ;
a2plusc2ovb2 =  (a^2 + c^2) / b^2; 


A0 = (1 + a2minc2ovb2)^2   -   4*((a*cos(gamma)/b)^2);
A1 = - a2minc2ovb2 * (1 + a2minc2ovb2) * cos(beta)     +    2 * ((a * cos(gamma) /  b)^2) * cos (beta)     -     (1 - a2plusc2ovb2) * cos(alpha) * cos(gamma);
A1 = 4 * A1;
A2 = a2minc2ovb2^2   -   1   +   2*((a2minc2ovb2 * cos(beta))^2)  +  2 *(  ((b^2 - c^2)/(b^2))  * (cos(alpha))^2  )   - 4*a2plusc2ovb2*cos(alpha)*cos(beta)*cos(gamma)   +   2*((b^2 - a^2)/(b^2))*((cos(gamma))^2);
A2 = 2* A2;
A3 = a2minc2ovb2 * (1 - a2minc2ovb2) * cos(beta)    -   (1 - a2plusc2ovb2) * cos(alpha) * cos(gamma)    +   2 * ((c * cos(alpha)/b)^2) * cos(beta);
A3 = 4 * A3;
A4 = (a2minc2ovb2 -1)^2   - (2 * c * cos(alpha) / b)^2;

%Solve polynomial
%instead of u and v for polynomial, use g and h - i.e., g = s2/s1 and h =
%s3/s1
p = [A4 A3 A2 A1 A0];
h = roots(p);
%choose only real roots - maybe this is not necessary?
h = h(imag(h)==0);
h = real(h);

%%%%%%%%%%%%%%%%%%%%%%%%%%%%%%%%%%%%%%%%%
%%%%%%%%%%%%%Find ray lengths

%For s1, which corresponds to sB. Should end up with 4 solns
%s_A =    (b^2) / (1 + h.^2  +  2*h*cos(beta)  )     ;
%s_A = s_A(s_A~=0);
%s_A = transpose(s_A);
%s_A = s_A.^0.5;


%Find s2, which corresponds to sC.
counter = 1;
for i = 1:numel(h)

    s_1 = (b^2) / (1 + (h(i)^2) - 2*h(i)*cos(beta));
    s_1 = sqrt(s_1);

    G2 = s_1^2;
    G1 = - 2 * (s_1^2) * cos(gamma);
    G0 = (s_1^2 -c^2);

    g = roots([G2 G1 G0]);
    g = g(imag(g)==0);
    g = real(g);

    %First, solve for s_C, since it only depends on h and s_A:

    for j = 1:numel(g)
        soln(counter, 1) = s_1 * g(j);
        soln(counter, 3) = s_1 * h(i);
        soln(counter, 2) = s_1; 
        counter = counter +1;
    end

end

== matlab function P3P_Grunert/Subsystem/For Each Subsystem/Custom P3P solver (Grunert)/MATLAB Function4 ==
  data: pnts_vectorsCameraCoords input; theta_raysABC_radians output
function theta_raysABC_radians = calcProjectionRayAngles(pnts_vectorsCameraCoords)

A_x_c = pnts_vectorsCameraCoords(:,1);
B_x_c = pnts_vectorsCameraCoords(:,2);
C_x_c = pnts_vectorsCameraCoords(:,3);

%theta_AB = acos(dot(A_x_c, B_x_c));
%theta_BC = acos(dot(B_x_c, C_x_c));
%theta_AC = acos(dot(C_x_c, A_x_c));

%theta_AB = atan2(norm(cross(A_x_c, B_x_c)), dot(A_x_c, B_x_c));
%theta_BC = atan2(norm(cross(B_x_c, C_x_c)), dot(B_x_c, C_x_c));
%theta_AC = atan2(norm(cross(A_x_c, C_x_c)), dot(A_x_c, C_x_c)); 

theta_AB = acos(dot(A_x_c, B_x_c)/(norm(A_x_c)*norm(B_x_c)));
theta_BC = acos(dot(B_x_c, C_x_c)/(norm(B_x_c)*norm(C_x_c)));
theta_AC = acos(dot(A_x_c, C_x_c)/(norm(A_x_c)*norm(C_x_c)));


theta_raysABC_radians = [theta_AB; theta_BC; theta_AC];

== matlab function P3P_Grunert/Subsystem/For Each Subsystem/extract P3P points and remove them from point matrices ==
  data: Vec_iterations input; x_ABC_i output size=[2,3]; X_pts_w input; X_ABC_w output size=[3,3]; x_pts_i input; x_rem_i output size=[60, 2]; X_rem_w output size=[60, 3]
function [x_ABC_i, X_ABC_w, x_rem_i, X_rem_w]= fcn(Vec_iterations, X_pts_w, x_pts_i)

num_pts = size(x_pts_i, 1);

%Initialise variables
rng("shuffle");
randNum1 = randi(num_pts);
randNum2 = randi(num_pts);
randNum3 = randi(num_pts);
while (randNum2 == randNum1)
    randNum2 = randi(num_pts);
end

while ((randNum3 ==randNum2) || (randNum3 == randNum1))
    randNum3 = randi(num_pts);
end
pnt1 = [X_pts_w(randNum1, :) x_pts_i(randNum1, :)];
pnt2 = [X_pts_w(randNum2, :) x_pts_i(randNum2, :)];
pnt3 = [X_pts_w(randNum3, :) x_pts_i(randNum3, :)];

%Choose random points  - sample until their x and y values are unique
% while (pnt1(1,1)==pnt2(1,1) || pnt1(1,1)==pnt3(1,1) || pnt2(1,1)==pnt3(1,1)) || (pnt1(1,2)==pnt2(1,2) || pnt1(1,2)==pnt3(1,2) || pnt2(1,2)==pnt3(1,2))
%     rng("shuffle");
%     randNum1 = randi(num_pts)
%     randNum2 = randi(num_pts)
%     randNum3 = randi(num_pts)
%     pnt1 = [X_pts_w(randNum1, :) x_pts_i(randNum1, :)];
%     pnt2 = [X_pts_w(randNum2, :) x_pts_i(randNum2, :)];
%     pnt3 = [X_pts_w(randNum3, :) x_pts_i(randNum3, :)];
% 
% end




%Force select the corner points
%randNums = [1 6 49];
%pnt1 = [X_pts_w(randNums(1, 1), :) x_pts_i(randNums(1, 1), :)];
%pnt2 = [X_pts_w(randNums(1, 2), :) x_pts_i(randNums(1, 2), :)];
%pnt3 = [X_pts_w(randNums(1, 3), :) x_pts_i(randNums(1, 3), :)];

%Remove training points from the list - i.e., develop "verification" set
X_rem_w = X_pts_w;
%X_rem_w((randNums(1)), :) = [];
%X_rem_w((randNums(2)-1), :) = [];
%X_rem_w((randNums(3)-2), :) = [];

x_rem_i = x_pts_i;
%x_rem_i(randNums(1), :) = [];
%x_rem_i((randNums(2)-1), :) = [];
%x_rem_i((randNums(3)-2), :) = [];


%Must put the points "in order" - is this necessary? Not sure. Early
%results suggest that it might be.
X_train = [pnt1; pnt2; pnt3];
X_train =sortrows(X_train, 2);          %sort by y-coordinate (world)
X_train_sorted = X_train;
%Swap rows
if X_train(2, 1) > X_train(3, 1)
    X_train_sorted([2 3], :) = X_train([3 2], :);
end

X_A_w = X_train_sorted(1, 1:3);
X_B_w = X_train_sorted(2, 1:3);
X_C_w = X_train_sorted(3, 1:3);

x_A_i = X_train_sorted(1, 4:5);
x_B_i = X_train_sorted(2, 4:5);
x_C_i = X_train_sorted(3, 4:5);

X_ABC_w_vert = [X_A_w; X_B_w; X_C_w];
X_ABC_w = transpose(X_ABC_w_vert);

x_ABC_i_vert = [x_A_i; x_B_i; x_C_i];
x_ABC_i = transpose(x_ABC_i_vert);

== matlab function P3P_Grunert/Subsystem/Custom P3P solver (Grunert)/Find ray lengths ==
  data: l_AB input; soln output size=[4, 3]; l_BC input; l_AC input; theta input
function soln = fcn(l_AB, l_BC, l_AC, theta)

soln = zeros(4, 3);


%Calculate polynomial coefficients
a = l_BC;
b = l_AC;
c = l_AB;

gamma = theta(3); %theta_AC
alpha = theta(2); %theta_BC
beta = theta(1); %theta_AB


a2minc2ovb2 =  (a^2 - c^2) / b^2 ;
a2plusc2ovb2 =  (a^2 + c^2) / b^2; 


A0 = (1 + a2minc2ovb2)^2   -   4*((a*cos(gamma)/b)^2);
A1 = - a2minc2ovb2 * (1 + a2minc2ovb2) * cos(beta)     +    2 * ((a * cos(gamma) /  b)^2) * cos (beta)     -     (1 - a2plusc2ovb2) * cos(alpha) * cos(gamma);
A1 = 4 * A1;
A2 = a2minc2ovb2^2   -   1   +   2*((a2minc2ovb2 * cos(beta))^2)  +  2 *(  ((b^2 - c^2)/(b^2))  * (cos(alpha))^2  )   - 4*a2plusc2ovb2*cos(alpha)*cos(beta)*cos(gamma)   +   2*((b^2 - a^2)/(b^2))*(cos(gamma)^2);
A2 = 2* A2;
A3 = a2minc2ovb2 * (1 - a2minc2ovb2) * cos(beta)    -   (1 - a2plusc2ovb2) * cos(alpha) * cos(gamma)    +   2 * ((c * cos(alpha)/b)^2) * cos(beta);
A3 = 4 * A3;
A4 = (a2minc2ovb2 -1)^2   - (2 * c * cos(alpha) / b)^2;

%Solve polynomial
%instead of u and v for polynomial, use g and h - i.e., g = s2/s1 and h =
%s3/s1
p = [A4 A3 A2 A1 A0];
h = roots(p);
%choose only real roots - maybe this is not necessary?
h = h(imag(h)==0);
h = real(h);

%%%%%%%%%%%%%%%%%%%%%%%%%%%%%%%%%%%%%%%%%
%%%%%%%%%%%%%Find ray lengths

%For s1, which corresponds to sA. Should end up with 4 solns
%s_A =    (b^2) / (1 + h.^2  +  2*h*cos(beta)  )     ;
%s_A = s_A(s_A~=0);
%s_A = transpose(s_A);
%s_A = s_A.^0.5;


%Find s2, which corresponds to sC.
counter = 1
for i = 1:numel(h)

    s_A = (b^2) / (1 + (h(i)^2) - 2*h(i)*cos(beta));
    s_A = sqrt(s_A);

    G2 = s_A^2;
    G1 = - 2 * (s_A^2) * cos(gamma);
    G0 = (s_A -c)^2;

    g = roots([G2 G1 G0]);
    g = g(imag(g)==0);
    g = real(g);

    %First, solve for s_C, since it only depends on h and s_A:

    for j = 1:numel(g)
        soln(counter, 1) = s_A;
        soln(counter, 3) = s_A * g(j);
        soln(counter, 2) = h(i) * s_A;
        counter = counter +1
    end

end

== matlab function P3P_Grunert/Subsystem/Image size calculator (in pixels) ==
  data: imageMatrix input; imageSize output
function imageSize = fcn(imageMatrix)

imageSize = [size(imageMatrix, 1) size(imageMatrix,2)];

== matlab function P3P_Grunert/Subsystem/MATLAB P3P solver1 ==
  data: estTransform input; K input; imagePts input; worldPts input; imageSize input; A_builtin output size=[4,4]; A_cust output size=[4,4]; Rt_builtin output size=[3,4]
function [A_builtin, A_cust, Rt_builtin]= fcn(estTransform, K, imagePts, worldPts, imageSize)

 %   imagePts_vert = transpose(imagePts);
 %   worldPts_vert = transpose(worldPts);
    focalLngth = [K(1,1) K(2,2)];
    principalPnt = [K(1,3) K(2,3)];
    maxError = 0.5; %mm

    coder.extrinsic('builtinP3P');
    A = zeros(4,4);
    A_cust = zeros(4,4);

    
    estTransform_R =estTransform(:, 1:3);
    estTransform_t =estTransform(:, 4);

    A = builtinP3P(imagePts, worldPts, focalLngth, principalPnt, imageSize, maxError, estTransform_t, estTransform_R, 0);
    A_builtin = A;
    Rt_builtin = A(1:3, 1:4);
    
    A_cust(1:3,1:4) = estTransform(1:3, 1:4);
    A_cust(4,:) = [0 0 0 1];

== matlab function P3P_Grunert/Subsystem/Outer corner selectors/MATLAB Function ==
  data: boardSize input; B_index output; C_index output; D_index output
function [B_index, C_index, D_index]= fcn(boardSize)

B_index = boardSize(1) - 1;
C_index = ((boardSize(1) - 1) * (boardSize(2) - 2)) + 1;
D_index = ((boardSize(1) - 1) * (boardSize(2) - 1)) ;

== matlab function P3P_Grunert/Subsystem/Outer corner selectors/Outer corner selector ==
  data: x_ABC_i output; x_D_i output; pntMatrix input; A_index input; B_index input; C_index input; D_index input
function [x_ABC_i, x_D_i] = fcn(pntMatrix, A_index, B_index, C_index, D_index)

%Obtain pixel positions
A_u = pntMatrix(A_index,1);
A_v = pntMatrix(A_index,2);

B_u = pntMatrix(B_index, 1);
B_v = pntMatrix(B_index, 2);

C_u = pntMatrix( C_index , 1);
C_v = pntMatrix( C_index , 2);

D_u = pntMatrix( D_index, 1);
D_v = pntMatrix(D_index, 2);


%Created augmented U matrices - i.e., add extra row of "1"
x_ABC_i = [A_u B_u C_u; A_v B_v C_v];
%pnts_U_ABC_aug = [pnts_U_ABC; 1 1 1];

%pnts_X_c = inv(K) * pnts_U_ABC_aug;

%pntVectors_cameraCoords = pnts_X_c;
%pntsABC_imageCoords = pnts_U_ABC;
%pntsABCD_imageCoords = [A_u B_u C_u D_u; A_v B_v C_v D_v];
x_D_i = [D_u; D_v];

== matlab function P3P_Grunert/Subsystem/Outer corner selectors/Outer corner selector (world frame) ==
  data: X_Pts_w input; X_ABC_w output size=[3, 3]; X_D_w output size=[3, 1]; A_index input; B_index input; C_index input; D_index input
function [X_ABC_w, X_D_w]= fcn(X_Pts_w, A_index, B_index, C_index, D_index)
    
    X_A_w = X_Pts_w(A_index, :);
    X_B_w = X_Pts_w(B_index, :);
    X_C_w = X_Pts_w(C_index, :);
    X_D_w_vert = X_Pts_w(D_index, :);

    X_ABC_w_vert = [X_A_w; X_B_w; X_C_w];
    X_ABC_w = transpose(X_ABC_w_vert);
    X_D_w = transpose(X_D_w_vert);

== matlab function P3P_Grunert/Subsystem/Project 4th point and calc reprojection error ==
  data: Rt input; K input; X_D_w input; x_D_i input; x_D_i_proj output size=[2,8]; soln output size=[3,4]; min_error output
function [x_D_i_proj, soln, min_error]= fcn(Rt, K, X_D_w, x_D_i)

%Calculate the projection of a fourth point onto the image plane, based on 
%the candidate rotation matrices and translation vectors. Later, we
%will check how well this corresponds with where it was actually observed.
    
    %Initialise vector
    x_D_i_proj = zeros(2,8); %where i stands for "image plane"
    x_D_i_proj_homo = zeros(3,8); %where i stands for "image plane"
    error = zeros(1,8);     %reprojection error
    soln = zeros(3, 4);

    %For each possible solution
    for n=1: size(Rt, 3)

        %Calculate projection of the point D
        x_D_i_proj_homo(:, n) = K * (  (Rt(:, 1:3, n) * X_D_w)  + Rt(:, 4,n)  );

        %Normalise by the 3rd dimension
        x_D_i_proj(1,n) = x_D_i_proj_homo(1,n)/x_D_i_proj_homo(3,n);
        x_D_i_proj(2,n) = x_D_i_proj_homo(2,n)/x_D_i_proj_homo(3,n);

        %Calculate reprojection error
        error(1, n) = norm(x_D_i - x_D_i_proj(:, n));
    
    end

    %Choose lower reprojection error
    error(1, 1) = norm(x_D_i - x_D_i_proj(:, 1));
    min_error = error(1,1);
    soln = Rt(:, :, 1);
    
    for j=2 : size(x_D_i_proj, 2)
        
        if error(1, j) < min_error
            min_error = error(1, j);
            soln = Rt(:, :, j);
        end
    
    end
